simulink model "PicontrollerMotor"  (R2023a)
settings: Solver=VariableStepAuto  StartTime=0.0  StopTime=10.0  RelTol=1e-3
model workspace (MAT data in the model file):
  J = 5e-05
  K = 0.2
  L = 0.01
  R = 4
  Sig = Simulink.Signal
  Sig.DataType = 'auto'
  Sig.Dimensions = -1
  Sig.DimensionsMode = 'auto'
  Sig.Complexity = 'auto'
  Sig.SampleTime = -1
  Sig.SamplingMode = 'auto'
  Ts = 0.01
  V = 7.4
  b = 0.0005
  ki = 7.33
  kp = 9.39
settings Model: Creator=MY PC  LastModifiedBy=MY PC

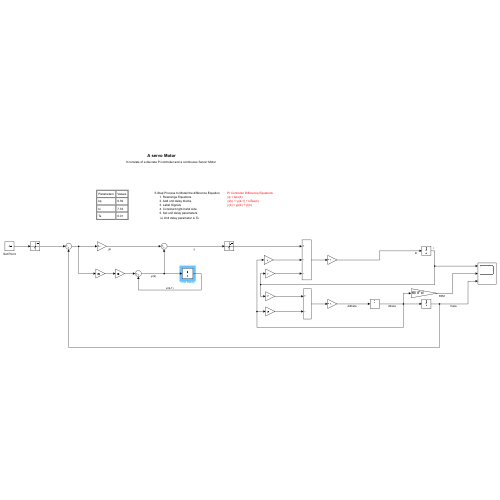
[thumbnail: Simulink's stored preview of the top-level diagram]
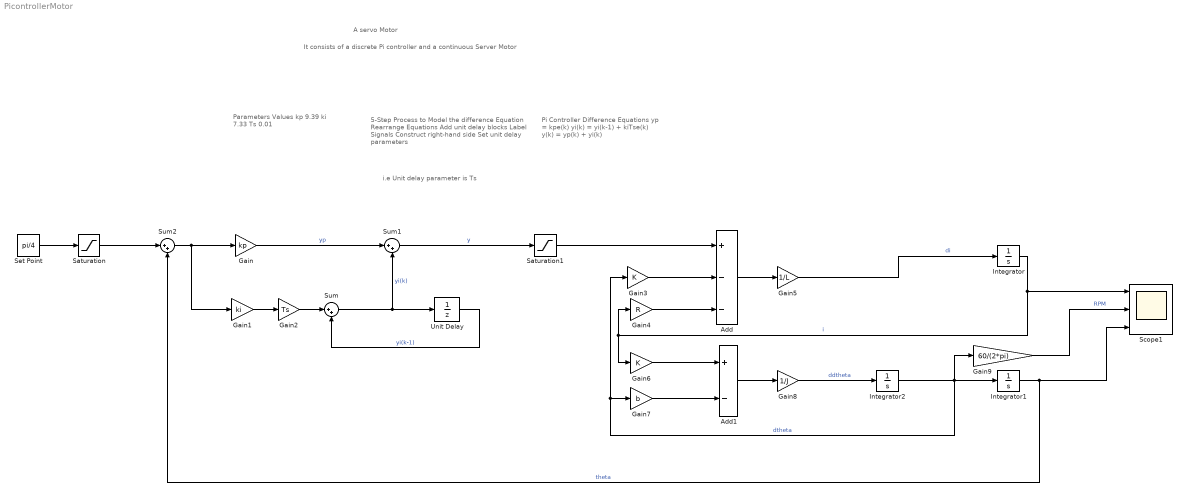
== system PicontrollerMotor ==
  note: It consists of a discrete Pi controller and a continuous Server Motor
  note: A servo Motor
  note: i.e Unit delay parameter is Ts
  note: 5-Step Process to Model the difference Equation
      | Rearrange Equations
      | Add unit delay blocks
      | Label Signals
      | Construct right-hand side
      | Set unit delay parameters
  note: Parameters
      | Values
      |
      | kp
      | 9.39
      |
      | ki
      | 7.33
      |
      | Ts
      | 0.01
  note: Pi Controller Difference Equations
      | yp = kpe(k)
      | yi(k) = yi(k-1) + kiTse(k)
      | y(k) = yp(k) + yi(k)
  Add : Sum  Inputs=+--
  Add1 : Sum  Inputs=+-
  Gain : Gain  Gain=kp
  Gain1 : Gain  Gain=ki
  Gain2 : Gain  Gain=Ts
  Gain3 : Gain  Gain=K
  Gain4 : Gain  Gain=R
  Gain5 : Gain  Gain=1/L
  Gain6 : Gain  Gain=K
  Gain7 : Gain  Gain=b
  Gain8 : Gain  Gain=1/J
  Gain9 : Gain  Gain=60/(2*pi)
  Integrator : Integrator
  Integrator1 : Integrator
  Integrator2 : Integrator
  Saturation : Saturate  UpperLimit=pi/4  LowerLimit=-pi/4
  Saturation1 : Saturate  UpperLimit=V  LowerLimit=-V
  Scope1 : Scope  NumInputPorts=3
  Set Point : Constant  Value=pi/4
  Sum : Sum  Inputs=|++
  Sum1 : Sum  Inputs=|++
  Sum2 : Sum  Inputs=|++
  Unit Delay : UnitDelay  SampleTime=Ts  HasFrameUpgradeWarning=on
  wires:
  Unit Delay/1 -> Sum/2  "yi(k-1)"
  Set Point/1 -> Saturation/1
  Gain/1 -> Sum1/1  "yp"
  Gain1/1 -> Gain2/1
  Gain2/1 -> Sum/1
  Sum/1 -> Sum1/2, Unit Delay/1  "yi(k)"
  Sum1/1 -> Saturation1/1  "y"
  Gain8/1 -> Integrator2/1  "ddtheta"
  Gain9/1 -> Scope1/2  "RPM"
  Add/1 -> Gain5/1
  Gain3/1 -> Add/2
  Gain6/1 -> Add1/1
  Gain4/1 -> Add/3
  Integrator2/1 -> Gain9/1, Gain7/1, Gain3/1, Integrator1/1  "dtheta"
  Gain7/1 -> Add1/2
  Gain5/1 -> Integrator/1  "di"
  Integrator1/1 -> Sum2/2, Scope1/3  "theta"
  Integrator/1 -> Scope1/1, Gain4/1, Gain6/1  "i"
  Add1/1 -> Gain8/1
  Sum2/1 -> Gain1/1, Gain/1
  Saturation1/1 -> Add/1
  Saturation/1 -> Sum2/1
